simulink model "qubeLQGR2"  (R2021b)
settings: Solver=ode1  StartTime=0.0  StopTime=50  RelTol=1e-3  EnableMultiTasking=on
values from neighbouring files (symbols this model uses):
  h = log(abs(sec(theta)+tan(theta))-C1*alpha)    [Design_of_nonlinear_controller.m]    (also in MPC_controller.m = 0.01; MPC_controller_withint_testing.m = 0.01)
undefined symbols (not defined in the file or in its folder): Humusoft, MF634
libraries: sldrtlib x2, simulink x2, eeGeneralControl x2, eeLuenbergerObserver x1
settings Model: Creator=rbabuska  LastModifiedBy=wpanijhuis
settings SolverCC: AlgebraicLoopSolver=TrustRegion
settings DataIOCC: LimitDataPoints=on  SaveFormat=Array  SignalLoggingSaveFormat=ModelDataLogs  ReturnWorkspaceOutputs=off
settings OptimizationCC: ExpressionDepthLimit=2147483647  LifeSpan=inf
settings DebuggingCC: UnderspecifiedInitializationDetection=Classic  MergeDetectMultiDrivingBlocksExec=none  FcnCallInpInsideContextMsg=warning  StateNameClashWarn=warning  SFUnexpectedBacktrackingDiag=warning  SFNoUnconditionalDefaultTransitionDiag=warning  SFExecutionAtInitializationDiag=none  SFMachineParentedDataDiag=warning  ArithmeticOperatorsInVariantConditions=warning
settings HardwareCC: ProdBitPerPointer=32  ProdBitPerSizeT=32  ProdBitPerPtrDiffT=32  ProdLargestAtomicFloat=None  ProdIntDivRoundTo=Undefined  ProdEndianess=Unspecified  ProdWordSize=32  ProdHWDeviceType=32-bit Generic
settings ModelReferenceCC: PropagateSignalLabelsOutOfModel=off
settings SFSimCC: SimUseLocalCustomCode=off  CustomCodeUndefinedFunction=UseInterfaceOnly
settings RTWCC: RTWUseLocalCustomCode=off
settings CodeAppCC: StateflowObjectComments=on
settings GRTTargetCC: TargetLangStandard=C89/C90 (ANSI)  CombineOutputUpdateFcns=off  GRTInterface=on
settings ConfigComp: CovMetricSettings=dw  CovSaveCumulativeToWorkspaceVar=on  CovSaveSingleToWorkspaceVar=on  CovExternalEMLEnable=off  CovSFcnEnable=off

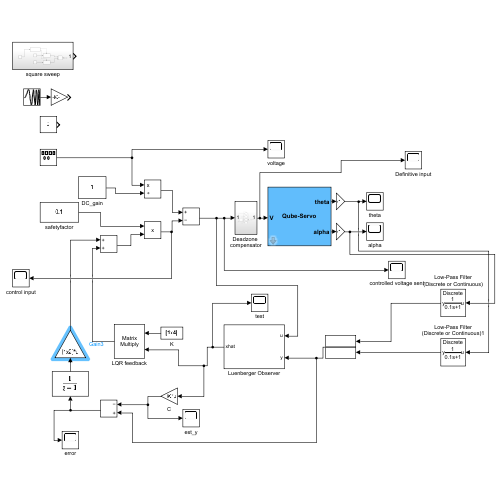
[thumbnail: Simulink's stored preview of the top-level diagram]
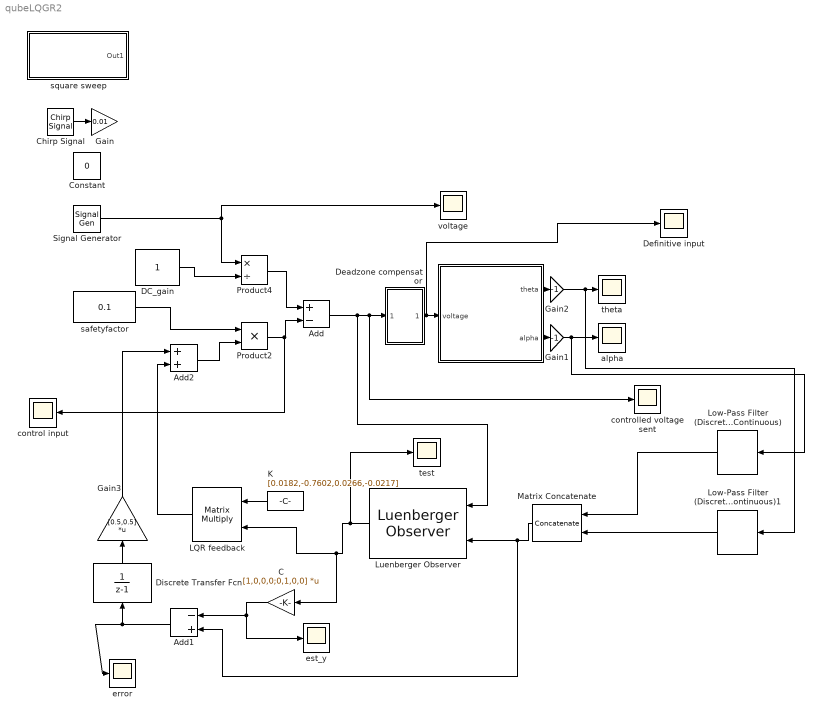
== system qubeLQGR2 ==
  " " : Subsystem  LoadFcn=hwinit  InitFcn=hwinit  mask{h=h}
      mask prompts: h "Sampling period [s]"
      mask Display:
      | disp('Qube-Servo')
      | port_label('output',1,'theta')
      | port_label('output',2,'alpha')
      | port_label('input',1,'V')
  Add : Sum  Inputs=+-
  Add1 : Sum  Inputs=-+
  Add2 : Sum
  C : Gain  Gain=[1,0,0,0;0,1,0,0]  Multiplication=Matrix(K*u)
  Chirp Signal : simulink/Sources/Chirp Signal  f1=4  T=50  f2=8
  Constant : Constant  Value=0
  DC_gain : Constant
  Deadzone compensator : Subsystem
  Definitive input : Scope
  Discrete Transfer Fcn : DiscreteTransferFcn  Denominator=[1 -1]
  Gain : Gain  Gain=0.01
  Gain1 : Gain  Gain=-1
  Gain2 : Gain  Gain=-1
  Gain3 : Gain  Gain=[0.5,0.5]  Multiplication=Matrix(K*u)
  K : Constant  Value=[0.0182,-0.7602,0.0266,-0.0217]  VectorParams1D=off
  LQR feedback : Product  Multiplication=Matrix(*)
  Low-Pass Filter (Discrete or Continuous) : eeGeneralControl/Low-Pass Filter (Discrete or Continuous)  K=1  T=0.1  B=inf  A=-inf  init_option=Inherited from block input  x0=0  Ts=-1
  Low-Pass Filter (Discrete or Continuous)1 : eeGeneralControl/Low-Pass Filter (Discrete or Continuous)  K=1  T=0.1  B=inf  A=-inf  init_option=Inherited from block input  x0=0  Ts=-1
  Luenberger Observer : eeLuenbergerObserver/Luenberger Observer  StateSpaceType=Discrete-time  Ad=[0.9988,0.00522,0.00985,0.00003514;0.001312,0.9887,0.00003652,0.009899;-0.2421,1.035,0.9698,0.008718;0.261,-2.255,0.007675,0.9761]  Bd=[0.05646;-0.05502;11.22;-10.95]  Cd=[1,0,0,0;0,1,0,0]  Dd=[0;0]  A=[0,0,1,0;0,0,0,1;-24.67,105.9,-2.944,0.3597;26.45,-228.2,0.6536,-1.271]  B=[0;0;1143;-1110]  C=[1,0,0,0;0,1,0,0]  D=[0;0]  ObserverDesign=Desired eigenvalues  Ld=1  DesiredEigenvalues=[-0.15, -0.16, -0.165, -0.17]  x0=[0;0;0;0]  Tsd=0.1  Ts=h
      settings: SourceProductBaseCode=PS
  Matrix Concatenate : Concatenate  ConcatenateDimension=2
  Product2 : Product
  Product4 : Product  Inputs=*/
  Signal Generator : SignalGenerator  WaveForm=square  Amplitude=0.00  Frequency=0.2
  alpha : Scope
  control input : Scope
  controlled voltage sent : Scope
  error : Scope
  est_y : Scope
  safetyfactor : Constant  Value=0.1
  square sweep : Subsystem
  test : Scope
  theta : Scope
  voltage : Scope
  wires:
  Gain2/1 -> Low-Pass Filter (Discrete or Continuous)1/1, theta/1
  Matrix Concatenate/1 -> Add1/2, Luenberger Observer/2
  K/1 -> LQR feedback/1
  Luenberger Observer/1 -> test/1, C/1, LQR feedback/2
  safetyfactor/1 -> Product2/1
  Product2/1 -> control input/1, Add/2
  DC_gain/1 -> Product4/2
  Product4/1 -> Add/1
  Deadzone compensator/1(Out1) -> Definitive input/1, " "/1(voltage)
  Low-Pass Filter (Discrete or Continuous)/1 -> Matrix Concatenate/1
  Gain1/1 -> Low-Pass Filter (Discrete or Continuous)/1, alpha/1
  Low-Pass Filter (Discrete or Continuous)1/1 -> Matrix Concatenate/2
  Signal Generator/1 -> voltage/1, Product4/1
  " "/2(alpha) -> Gain1/1
  " "/1(theta) -> Gain2/1
  Add/1 -> Luenberger Observer/1, controlled voltage sent/1, Deadzone compensator/1(In1)
  Chirp Signal/1 -> Gain/1
  C/1 -> Add1/1, est_y/1
  Add1/1 -> error/1, Discrete Transfer Fcn/1
  Discrete Transfer Fcn/1 -> Gain3/1
  Add2/1 -> Product2/2
  LQR feedback/1 -> Add2/2
  Gain3/1 -> Add2/1

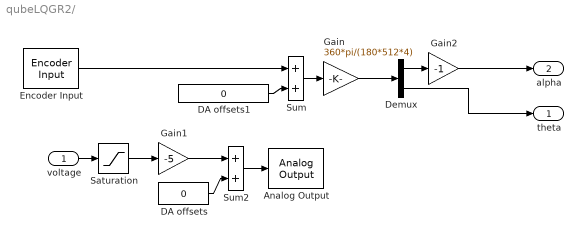
== system qubeLQGR2/  ==
  voltage : Inport
  Analog Output : sldrtlib/Analog Output  SampleTime=h  MaxMissedTicks=100  ShowMissedTicks=off  YieldWhenWaiting=off  DrvName=Humusoft/MF634  DrvAddress=4294967295  DrvOptions=0  Channels=[1]  RangeMode=2  VoltRange=1  InitialValue=0  FinalValue=0
      settings: AttributesFormatString=Humusoft\nMF634 [auto]
  DA offsets : Constant  Value=0
  DA offsets1 : Constant  Value=0  SampleTime=h
  Demux : Demux  Outputs=2
  Encoder Input : sldrtlib/Encoder Input  SampleTime=h  MaxMissedTicks=100  ShowMissedTicks=off  YieldWhenWaiting=off  DrvName=Humusoft/MF634  DrvAddress=4294967295  DrvOptions=0  Channels=[1,2]  QuadMode=3  IndexPulse=1  InputFilter=Inf  DataType=1
      settings: AttributesFormatString=Humusoft\nMF634 [auto]
  Gain : Gain  Gain=360*pi/(180*512*4)  SaturateOnIntegerOverflow=on  OutDataTypeStr=Inherit: Same as input  ParamDataTypeStr=Inherit: Same as input
  Gain1 : Gain  Gain=-5  SaturateOnIntegerOverflow=on  OutDataTypeStr=Inherit: Same as input  ParamDataTypeStr=Inherit: Same as input
  Gain2 : Gain  Gain=-1  SaturateOnIntegerOverflow=on  OutDataTypeStr=Inherit: Same as input  ParamDataTypeStr=Inherit: Same as input
  Saturation : Saturate  UpperLimit=1  LowerLimit=-1
  Sum : Sum  InputSameDT=on  SaturateOnIntegerOverflow=on  OutDataTypeStr=Inherit: Same as first input
  Sum2 : Sum  InputSameDT=on  SaturateOnIntegerOverflow=on  OutDataTypeStr=Inherit: Same as first input
  theta : Outport  Tag=Cable length
  alpha : Outport  Tag=Cable length  Port=2
  wires:
  Sum/1 -> Gain/1
  DA offsets1/1 -> Sum/2
  Gain1/1 -> Sum2/1
  Sum2/1 -> Analog Output/1
  DA offsets/1 -> Sum2/2
  voltage/1 -> Saturation/1
  Encoder Input/1 -> Sum/1
  Saturation/1 -> Gain1/1
  Demux/1 -> Gain2/1
  Gain/1 -> Demux/1
  Gain2/1 -> alpha/1
  Demux/2 -> theta/1

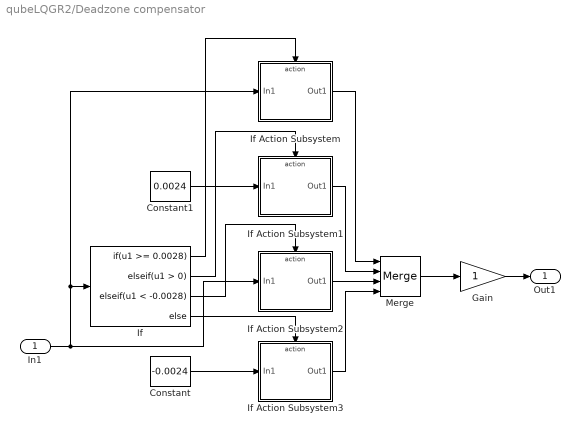
== system qubeLQGR2/Deadzone compensator ==
  In1 : Inport
  Constant : Constant  Value=-0.0024
  Constant1 : Constant  Value=0.0024
  Gain : Gain
  If : If  IfExpression=u1 >= 0.0028  ElseIfExpressions=u1 > 0, u1 < -0.0028
  If Action Subsystem : Subsystem  TreatAsAtomicUnit=on
  If Action Subsystem1 : Subsystem  TreatAsAtomicUnit=on
  If Action Subsystem2 : Subsystem  TreatAsAtomicUnit=on
  If Action Subsystem3 : Subsystem  TreatAsAtomicUnit=on
  Merge : Merge  Inputs=4
  Out1 : Outport
  wires:
  If Action Subsystem/1(Out1) -> Merge/1
  Gain/1 -> Out1/1
  If/4 -> If Action Subsystem3/Action
  If Action Subsystem2/1(Out1) -> Merge/3
  If/3 -> If Action Subsystem2/Action
  Merge/1 -> Gain/1
  If/2 -> If Action Subsystem1/Action
  Constant1/1 -> If Action Subsystem1/1(In1)
  If/1 -> If Action Subsystem/Action
  Constant/1 -> If Action Subsystem3/1(In1)
  If Action Subsystem3/1(Out1) -> Merge/4
  If Action Subsystem1/1(Out1) -> Merge/2
  In1/1 -> If Action Subsystem/1(In1), If/1, If Action Subsystem2/1(In1)

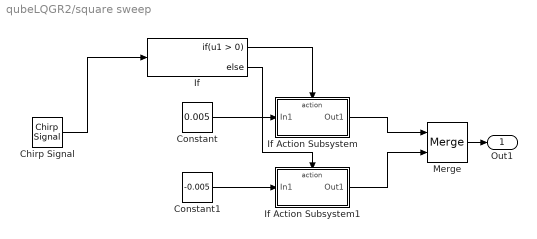
== system qubeLQGR2/square sweep ==
  Chirp Signal : simulink/Sources/Chirp Signal  f1=0  T=120  f2=5
  Constant : Constant  Value=0.005
  Constant1 : Constant  Value=-0.005
  If : If
  If Action Subsystem : Subsystem  TreatAsAtomicUnit=on
  If Action Subsystem1 : Subsystem  TreatAsAtomicUnit=on
  Merge : Merge
  Out1 : Outport
  wires:
  Merge/1 -> Out1/1
  If/2 -> If Action Subsystem1/Action
  Chirp Signal/1 -> If/1
  Constant/1 -> If Action Subsystem/1(In1)
  If Action Subsystem1/1(Out1) -> Merge/2
  If Action Subsystem/1(Out1) -> Merge/1
  If/1 -> If Action Subsystem/Action
  Constant1/1 -> If Action Subsystem1/1(In1)

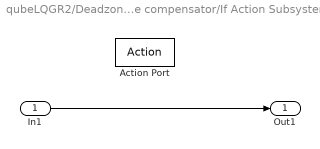
== system qubeLQGR2/Deadzone compensator/If Action Subsystem ==
  In1 : Inport
  Action Port : ActionPort  ActionPortLabel=if(u1 >= 0.0028)
  Out1 : Outport
  wires:
  In1/1 -> Out1/1

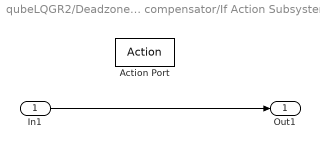
== system qubeLQGR2/Deadzone compensator/If Action Subsystem1 ==
  In1 : Inport
  Action Port : ActionPort  ActionPortLabel=elseif(u1 > 0)
  Out1 : Outport
  wires:
  In1/1 -> Out1/1

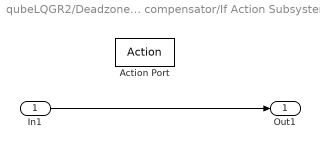
== system qubeLQGR2/Deadzone compensator/If Action Subsystem2 ==
  In1 : Inport
  Action Port : ActionPort  ActionPortLabel=elseif( u1 < -0.0028)
  Out1 : Outport
  wires:
  In1/1 -> Out1/1

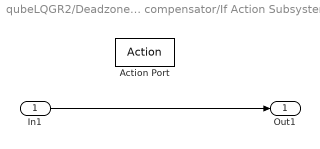
== system qubeLQGR2/Deadzone compensator/If Action Subsystem3 ==
  In1 : Inport
  Action Port : ActionPort  ActionPortLabel=else
  Out1 : Outport
  wires:
  In1/1 -> Out1/1

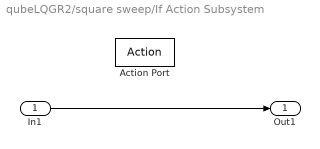
== system qubeLQGR2/square sweep/If Action Subsystem ==
  In1 : Inport
  Action Port : ActionPort  ActionPortLabel=if(u1 > 0)
  Out1 : Outport
  wires:
  In1/1 -> Out1/1

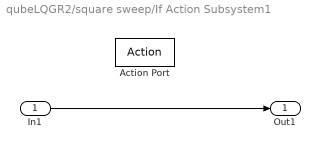
== system qubeLQGR2/square sweep/If Action Subsystem1 ==
  In1 : Inport
  Action Port : ActionPort  ActionPortLabel=else
  Out1 : Outport
  wires:
  In1/1 -> Out1/1
